simulink model "hardware_sim_rectifier_buck"  (R2023b)
settings: Solver=VariableStepAuto  StartTime=0.0  StopTime=0.2  MaxStep=1e-6  RelTol=1e-3
libraries: spsSeriesRLCBranchLib x9, spsVoltageMeasurementLib x8, spsDiodeLib x7, spsCurrentMeasurementLib x6, spsACVoltageSourceLib x3, spsMeanLib x2, spsDCVoltageSourceLib x1, spsGroundLib x1, spsMosfetLib x1, sps_lib x1
settings Model: Creator=elife  LastModifiedBy=elife
settings DataIOCC: ReturnWorkspaceOutputs=off

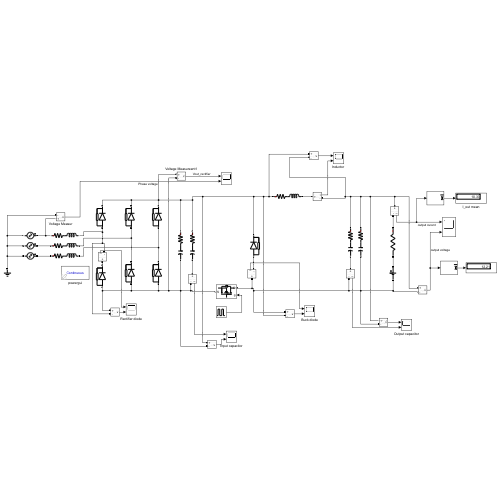
[thumbnail: Simulink's stored preview of the top-level diagram]
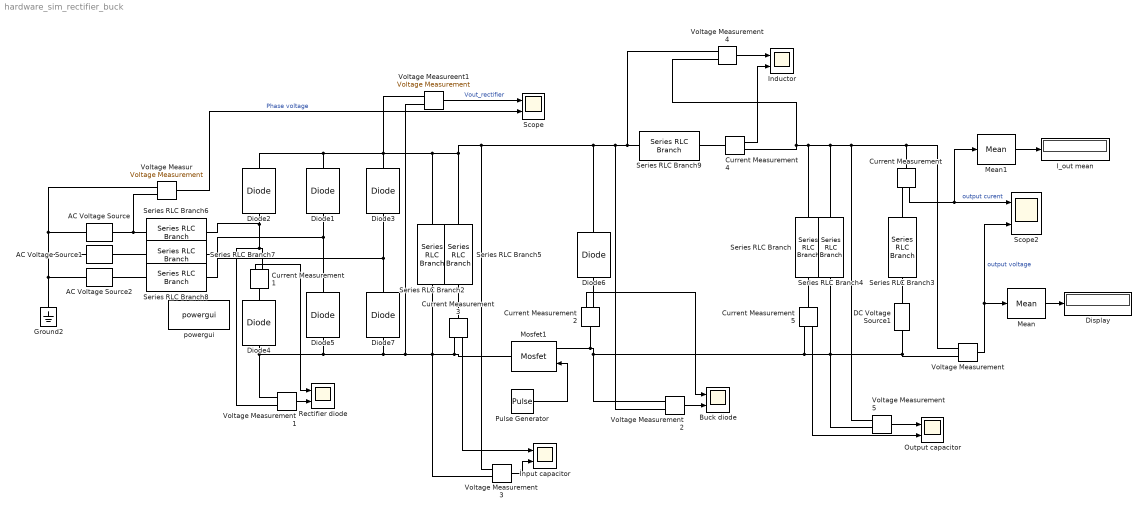
== system hardware_sim_rectifier_buck ==
  AC Voltage Source : spsACVoltageSourceLib/AC Voltage Source  Amplitude=25*sqrt(2)/sqrt(3)  Phase=0  Frequency=50  SampleTime=0  Measurements=None  BusType=swing  Pref=10e3  Qref=0  Qmin=-inf  Qmax=+inf
  AC Voltage Source1 : spsACVoltageSourceLib/AC Voltage Source  Amplitude=25*sqrt(2)/sqrt(3)  Phase=120  Frequency=50  SampleTime=0  Measurements=None  BusType=swing  Pref=10e3  Qref=0  Qmin=-inf  Qmax=+inf
  AC Voltage Source2 : spsACVoltageSourceLib/AC Voltage Source  Amplitude=25*sqrt(2)/sqrt(3)  Phase=240  Frequency=50  SampleTime=0  Measurements=None  BusType=swing  Pref=10e3  Qref=0  Qmin=-inf  Qmax=+inf
  Buck diode : Scope  NumInputPorts=2
  Current Measurement{,1..5} (6 alike) : spsCurrentMeasurementLib/Current Measurement  PhasorSimulation=off  OutputType=Complex  PSBequivalent=0
  DC Voltage Source1 : spsDCVoltageSourceLib/DC Voltage Source  Amplitude=12  Measurements=None
  Diode{1..5,7} (6 alike) : spsDiodeLib/Diode  Ron=0.013  Lon=0  Vf=0.7  IC=0  UseSnubber=0  Rs=1.5  Cs=1.7e-7  Measurements=off
  Diode6 : spsDiodeLib/Diode  Ron=0.013  Lon=0  Vf=0.7  IC=0  UseSnubber=0  Rs=2.4  Cs=7.7e-8  Measurements=off
  Display : Display
  Ground2 : spsGroundLib/Ground  LConnTagsString=a
  I_out mean : Display
  "Inductor " : Scope  NumInputPorts=2
  Mean : spsMeanLib/Mean  Freq=60  Vinit=0  Ts=0
  Mean1 : spsMeanLib/Mean  Freq=60  Vinit=0  Ts=0
  Mosfet1 : spsMosfetLib/Mosfet  Ron=0.013  Lon=0  Rd=0.013  Vfd=0.7  IC=0  Rs=2  Cs=1.7e-7  Measurements=off
  Output capacitor : Scope  NumInputPorts=2
  Pulse Generator : DiscretePulseGenerator  PulseType=Time based  Period=1/10000  PulseWidth=38.8
  Rectifier diode : Scope  NumInputPorts=2
  Scope : Scope  NumInputPorts=2
  Scope2 : Scope  NumInputPorts=2
  Series RLC Branch : spsSeriesRLCBranchLib/Series RLC Branch  LConnTagsString=__new0  RConnTagsString=__new0  BranchType=RC  Resistance=0.08  Inductance=1e-3  SetiL0=off  InitialCurrent=0  Capacitance=470e-6  Setx0=off  InitialVoltage=0  Measurements=None
  Series RLC Branch2 : spsSeriesRLCBranchLib/Series RLC Branch  LConnTagsString=__new0  RConnTagsString=__new0  BranchType=RC  Resistance=0.08  Inductance=1e-3  SetiL0=off  InitialCurrent=0  Capacitance=680e-6  Setx0=off  InitialVoltage=0  Measurements=None
  Series RLC Branch3 : spsSeriesRLCBranchLib/Series RLC Branch  LConnTagsString=__new0  RConnTagsString=__new0  BranchType=R  Resistance=20e-3  Inductance=1e-3  SetiL0=off  InitialCurrent=0  Capacitance=680e-6  Setx0=off  InitialVoltage=0  Measurements=None
  Series RLC Branch4 : spsSeriesRLCBranchLib/Series RLC Branch  LConnTagsString=__new0  RConnTagsString=__new0  BranchType=RC  Resistance=0.08  Inductance=1e-3  SetiL0=off  InitialCurrent=0  Capacitance=470e-6  Setx0=off  InitialVoltage=0  Measurements=None
  Series RLC Branch5 : spsSeriesRLCBranchLib/Series RLC Branch  LConnTagsString=__new0  RConnTagsString=__new0  BranchType=RC  Resistance=0.08  Inductance=1e-3  SetiL0=off  InitialCurrent=0  Capacitance=680e-6  Setx0=off  InitialVoltage=0  Measurements=None
  Series RLC Branch6 : spsSeriesRLCBranchLib/Series RLC Branch  LConnTagsString=__new0  RConnTagsString=__new0  BranchType=RL  Resistance=5e-6  Inductance=1e-4  SetiL0=off  InitialCurrent=0  Capacitance=1e-6  Setx0=off  InitialVoltage=0  Measurements=None
  Series RLC Branch7 : spsSeriesRLCBranchLib/Series RLC Branch  LConnTagsString=__new0  RConnTagsString=__new0  BranchType=RL  Resistance=5e-6  Inductance=1e-4  SetiL0=off  InitialCurrent=0  Capacitance=1e-6  Setx0=off  InitialVoltage=0  Measurements=None
  Series RLC Branch8 : spsSeriesRLCBranchLib/Series RLC Branch  LConnTagsString=__new0  RConnTagsString=__new0  BranchType=RL  Resistance=5e-6  Inductance=1e-4  SetiL0=off  InitialCurrent=0  Capacitance=1e-6  Setx0=off  InitialVoltage=0  Measurements=None
  Series RLC Branch9 : spsSeriesRLCBranchLib/Series RLC Branch  LConnTagsString=__new0  RConnTagsString=__new0  BranchType=RL  Resistance=5e-3  Inductance=680e-6  SetiL0=off  InitialCurrent=0  Capacitance=1e-6  Setx0=off  InitialVoltage=0  Measurements=None
  Voltage Measur : spsVoltageMeasurementLib/Voltage Measurement  PhasorSimulation=off  OutputType=Complex  PSBequivalent=0
  Voltage Measureent1 : spsVoltageMeasurementLib/Voltage Measurement  PhasorSimulation=off  OutputType=Complex  PSBequivalent=0
  Voltage Measurement{,1..5} (6 alike) : spsVoltageMeasurementLib/Voltage Measurement  PhasorSimulation=off  OutputType=Complex  PSBequivalent=0
  powergui : sps_lib/powergui  Priority=1  SimulationMode=Continuous  SampleTime=50e-6  frequency=60  Iterations=50  frequencyindice=50  Pbase=100e6  ErrMax=1e-4  UnitsV=kV  UnitsW=MW  buscounter=0  FunctionMessages=off  echomessages=off  EnableUseOfTLC=off  CurrentSourceSwitches=off  DisableSnubberDevices=off  DisableRonSwitches=off  DisableVfSwitches=off  DisplayEquations=off  AutomaticDiscreteSolvers=off  SolverType=Tustin/Backward Euler (TBE)  Interpol=off  ExternalGateDelay=off  methode=off  Ts=100  x0status=blocks  SPID=on  SwTol=0  HookPort=off  NonlinearTolerance=1e-4  nMaxIteration=100  ContinueOnMaxIteration=off  RestoreLinks=warning  ResistiveCurrentMeasurement=off  Frange=[0:2:500]  Ylog=off  Xlog=on  ShowGrid=off  save=off  variable=ZData  structure=0  ZoomFFT=off  StartTime=0.0  cycles=1  DisplayStyle=1  fundamental=60  FreqAxis=off  MaxFrequency=1000  frequencyindicesteady=1  RmsSteady=1  display=off
  İnput capacitor : Scope  NumInputPorts=2
  wires:
  Voltage Measurement/1 -> Scope2/2, Mean/1  "output voltage"
  Mean/1 -> Display/1
  Current Measurement/1 -> Mean1/1, Scope2/1  "output curent"
  Voltage Measureent1/1 -> Scope/1  "Vout_rectifier"
  Voltage Measur/1 -> Scope/2  "Phase voltage"
  Pulse Generator/1 -> Mosfet1/1
  Mean1/1 -> I_out mean/1
  Current Measurement1/1 -> Rectifier diode/1
  Voltage Measurement1/1 -> Rectifier diode/2
  Current Measurement2/1 -> Buck diode/1
  Voltage Measurement2/1 -> Buck diode/2
  Current Measurement3/1 -> İnput capacitor/1
  Voltage Measurement3/1 -> İnput capacitor/2
  Current Measurement4/1 -> "Inductor "/2
  Voltage Measurement4/1 -> "Inductor "/1
  Current Measurement5/1 -> Output capacitor/2
  Voltage Measurement5/1 -> Output capacitor/1
  connections:
  AC Voltage Source2/LConn1 -- Ground2/LConn1 -- Voltage Measur/LConn2 -- AC Voltage Source/LConn1 -- AC Voltage Source1/LConn1
  Voltage Measurement/LConn1 -- Voltage Measurement5/LConn1 -- Current Measurement4/RConn1 -- Voltage Measurement4/LConn2 -- Series RLC Branch/LConn1 -- Series RLC Branch4/LConn1 -- Current Measurement/LConn1
  Series RLC Branch3/LConn1 -- Current Measurement/RConn1
  Series RLC Branch6/RConn1 -- Voltage Measurement1/LConn2 -- Current Measurement1/RConn1 -- Diode2/LConn1
  Series RLC Branch7/RConn1 -- Diode5/RConn1 -- Diode1/LConn1
  Series RLC Branch8/RConn1 -- Diode7/RConn1 -- Diode3/LConn1
  Series RLC Branch3/RConn1 -- DC Voltage Source1/RConn1
  Mosfet1/RConn1 -- Current Measurement3/RConn1 -- Voltage Measurement3/LConn2 -- Diode7/LConn1 -- Diode4/LConn1 -- Voltage Measurement1/LConn1 -- Diode5/LConn1 -- Voltage Measureent1/LConn2 -- Series RLC Branch2/RConn1
  Series RLC Branch6/LConn1 -- AC Voltage Source/RConn1 -- Voltage Measur/LConn1
  Series RLC Branch7/LConn1 -- AC Voltage Source1/RConn1
  Series RLC Branch8/LConn1 -- AC Voltage Source2/RConn1
  Current Measurement4/LConn1 -- Series RLC Branch9/RConn1
  Series RLC Branch2/LConn1 -- Voltage Measurement3/LConn1 -- Diode6/RConn1 -- Voltage Measurement2/LConn2 -- Voltage Measurement4/LConn1 -- Series RLC Branch9/LConn1 -- Series RLC Branch5/LConn1 -- Diode3/RConn1 -- Diode2/RConn1 -- Diode1/RConn1 -- Voltage Measureent1/LConn1
  Voltage Measurement5/LConn2 -- DC Voltage Source1/LConn1 -- Voltage Measurement/LConn2 -- Series RLC Branch4/RConn1 -- Current Measurement5/RConn1 -- Mosfet1/LConn1 -- Current Measurement2/LConn1 -- Voltage Measurement2/LConn1
  Current Measurement1/LConn1 -- Diode4/RConn1
  Current Measurement2/RConn1 -- Diode6/LConn1
  Current Measurement3/LConn1 -- Series RLC Branch5/RConn1
  Current Measurement5/LConn1 -- Series RLC Branch/RConn1
